simulink model "Test_Sim"  (R2020b)
settings: Solver=VariableStepAuto  StartTime=0.0  StopTime=inf  RelTol=1e-3
settings Model: Creator=FadliAziz  LastModifiedBy=FadliAziz

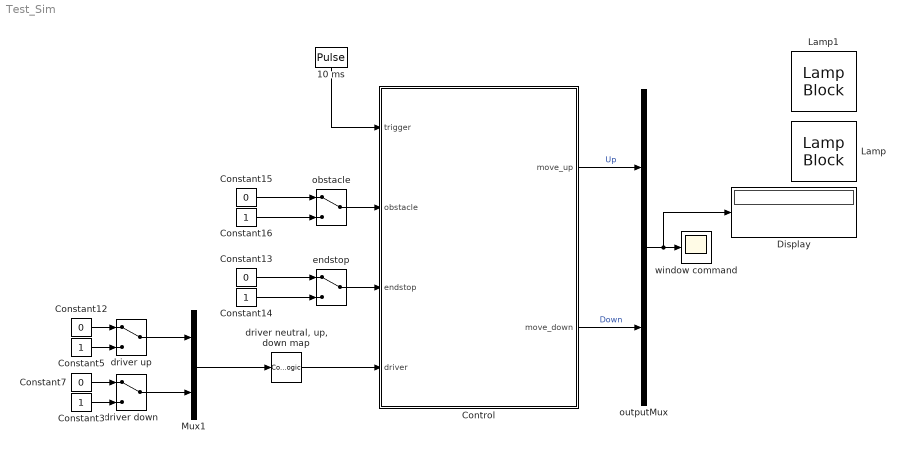
== system Test_Sim ==
  10 ms : DiscretePulseGenerator  SampleTime=10e-3
  Constant{7,12..13,15} (4 alike) : Constant  Value=0  OutDataTypeStr=boolean
  Constant{3,5,14,16} (4 alike) : Constant  OutDataTypeStr=boolean
  Control : Subsystem
  Display : Display
  Lamp : LampBlock
  Lamp1 : LampBlock
  Mux1 : Mux  Inputs=2
  "driver neutral, up, down map" : CombinatorialLogic  TruthTable=[1 0 0;0 0 1;0 1 0;1 0 0]
  driver down : ManualSwitch
  driver up : ManualSwitch
  endstop : ManualSwitch
  obstacle : ManualSwitch
  outputMux : Mux  Inputs=2
  window command : Scope
  wires:
  obstacle/1 -> Control/2(obstacle)
  Constant15/1 -> obstacle/1
  10 ms/1 -> Control/1(trigger)
  driver up/1 -> Mux1/1
  Mux1/1 -> "driver neutral, up, down map"/1
  Constant13/1 -> endstop/1
  Constant14/1 -> endstop/2
  endstop/1 -> Control/3(endstop)
  outputMux/1 -> Display/1, window command/1
  "driver neutral, up, down map"/1 -> Control/4(driver)
  Control/2(move_down) -> outputMux/2  "Down"
  Constant5/1 -> driver up/2
  Control/1(move_up) -> outputMux/1  "Up"
  Constant3/1 -> driver down/2
  Constant7/1 -> driver down/1
  driver down/1 -> Mux1/2
  Constant12/1 -> driver up/1
  Constant16/1 -> obstacle/2

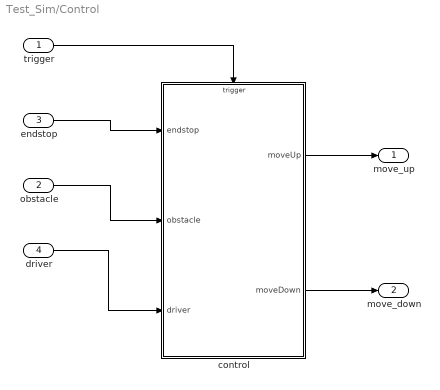
== system Test_Sim/Control ==
  trigger : Inport  OutDataTypeStr=double  Unit=sec  PortDimensions=1  SampleTime=0.01
  obstacle : Inport  Port=2  OutDataTypeStr=boolean  Unit=1  PortDimensions=1
  endstop : Inport  Port=3  OutDataTypeStr=boolean  Unit=1  PortDimensions=1
  driver : Inport  Port=4  OutDataTypeStr=boolean  Unit=1  PortDimensions=3
  control : Stateflow chart  TreatAsAtomicUnit=on
  move_up : Outport  OutDataTypeStr=boolean  Unit=1  PortDimensions=1  VectorParamsAs1DForOutWhenUnconnected=off
  move_down : Outport  Port=2  OutDataTypeStr=boolean  Unit=1  PortDimensions=1  VectorParamsAs1DForOutWhenUnconnected=off
  wires:
  driver/1 -> control/3(driver)
  trigger/1 -> control/Trigger
  endstop/1 -> control/1(endstop)
  control/1(moveUp) -> move_up/1
  obstacle/1 -> control/2(obstacle)
  control/2(moveDown) -> move_down/1

== stateflow chart Test_Sim/Control/control ==
  settings: executeAtInitialization=1
  state safe
    state driverNeutral
      entry:
      moveUp = 0;
      moveDown = 0;
    state driverDown
      entry: moveDown = 1;
      exit: moveDown = 0;
      state iniDriverDown
      state autoDriverDown
      state DriverDown
      iniDriverDown -> (junction 56) : after(100,ticks)
      (junction 56) -> autoDriverDown [order 1] : [driver[1]]
      (junction 56) -> DriverDown [order 2]
    state driverUp
      entry: moveUp = 1;
      exit: moveUp = 0;
      state iniDriverUp
      state DriverUp
      state autoDriverUp
      iniDriverUp -> (junction 57) : after(100,ticks)
      (junction 57) -> DriverUp [order 2]
      (junction 57) -> autoDriverUp [order 1] : [driver[1]]
    (default) -> driverNeutral
    driverNeutral -> iniDriverDown [order 2] : [driver[3]]
    DriverDown -> driverNeutral : [driver[1]]
    driverDown -> driverNeutral [order 1] : [endstop]
    DriverUp -> driverNeutral : [driver[1]]
    driverUp -> driverNeutral [order 2] : [endstop]
    driverNeutral -> iniDriverUp [order 1] : [driver[2]]
    driverDown -> DriverUp [order 2] : [driver[2]]
    driverUp -> DriverDown [order 1] : [driver[3]]
  state emergencyDown
    entry:
    moveUp = 0;
    moveDown = 1;
  (default) -> safe
  emergencyDown -> driverNeutral : [endstop | after(100,ticks)]
  safe -> emergencyDown : [obstacle]
  data: moveUp output boolean; moveDown output boolean; endstop input boolean; obstacle input boolean; driver input boolean size=3
  events: ticks input EITHER_EDGE_EVENT
